simulink model "test_emplanner_cs"  (R2021a)
settings: Solver=ode5  StartTime=0.0  StopTime=120  FixedStep=1/1000  RelTol=1e-3
PreLoadFcn:
  | mbxruntime.callbacks.PreLoadFcn(bdroot);
PostLoadFcn:
  | mbxruntime.callbacks.PostLoadFcn(bdroot);
InitFcn:
  | mbxruntime.callbacks.InitFcn(bdroot);
StartFcn:
  | mbxruntime.callbacks.StartFcn(bdroot);
StopFcn:
  | mbxruntime.callbacks.StopFcn(bdroot);
model workspace (MAT data in the model file):
  mbox_table : object (value not decoded)
  model_closed = 0
  sim_status = 0
values from neighbouring files (symbols this model uses):
  c_factor = 43.75    [emplanner_init.m]
  cf = -175016    [emplanner_init.m]
  cr = -130634    [emplanner_init.m]
  global_path_x = [-2.7494 -1.75001774493 -0.751894634419 0.244952249347 1.24051712279 2.23479835808 3.22779585569 4.21951007764 5.20994169183 6.19909144113 7.18696009523 8.17354843293 ... (3001 elements, 3001x1)]    [global_path.mat]
  global_path_y = [18.2589 18.2589 18.2589 18.2589 18.2589 18.2589 18.2589 18.2589 18.2589 18.2589 18.2589 18.2589 ... (3001 elements, 3001x1)]    [global_path.mat]
  KD_PID_distance = 0.0    (= 0)    [emplanner_init.m]
  KD_PID_speed = 0    [emplanner_init.m]
  KI_PID_distance = 0.0    (= 0)    [emplanner_init.m]
  KI_PID_speed = 0    [emplanner_init.m]
  KP_PID_distance = 0.5    [emplanner_init.m]
  KP_PID_speed = 1.8    [emplanner_init.m]
  la = 1.265    [emplanner_init.m]
  lb = 2.947-1.265    (= 1.682)    [emplanner_init.m]
  LQR_K1 = k(:,1)'    [emplanner_init.m]
  LQR_K2 = k(:,2)'    [emplanner_init.m]
  LQR_K3 = k(:,3)'    [emplanner_init.m]
  LQR_K4 = k(:,4)'    [emplanner_init.m]
  m = 2020    [emplanner_init.m]
  rack_displacement = [-39.14 , -37.2 , -35.29 , -33.43 , -31.6 , -29.81 , -28.06 , -26.34 , -24.66 ,      -23.01 , -21.38 , -19.79 , -18.23 , -16.69 , -15.18 , -13.7 , -12.23 , -10.8 , -9.38 , -7.98 ,     -6.61 , -5.25 , -3.91 , -2.59 , -1.29 , 0 , 1.27 , 2.54 , 3.78 , 5.02 , 6.24 , 7.46 , 8.66 ,      9.86 , 11.05 , 12.24 , 13.41 , 14.59 , 15.76 , 16.92 , 18.09 , 19.25 , 20.42 , 21.59 , 22.76 ,      23.93 , 25.11 , 26 ...(+26 chars)    [emplanner_init.m]
  right_wheel_ground = [-70 ,-67.2 , -64.4 , -61.6 , -58.8 , -56 , -53.2 , -50.4 , -47.6 , -44.8 , -42 ,      -39.2 , -36.4 , -33.6 , -30.8 , -28 , -25.2 , -22.4 , -19.6 , -16.8 , -14 , -11.2 , -8.4 , -5.6 ,      -2.8 , 0 , 2.8 , 5.6 , 8.4 , 11.2 , 14 , 16.8 , 19.6 , 22.4 , 25.2 , 28 , 30.8 , 33.6 , 36.4 ,      39.2 , 42 , 44.8 , 47.6 , 50.4 , 53.2 , 56 , 58.8 , 61.6 , 64.4 , 67.2 , 70 ]    [emplanner_init.m]
  vx_break_point = zeros(1,5000)    [emplanner_init.m]
undefined symbols (not defined in the file or in its folder): aubr, DiscIntNeverNeededParam, tablebr, vubr, warningInitialVelocity, x0
libraries: PreScanSimulinkLibrary x27, simulink x19, simulink_extras x6, Solver_SF x1
(part 10 of 11)

== matlab function test_emplanner_cs/Audi_A8_Sedan_1/decision&planning module/EM Planner/obs/cartesian2frenet1/MATLAB Function1 ==
  data: x_set input; s_set output; y_set input; frenet_path_x input; frenet_path_y input; proj_x_set input; proj_y_set input; proj_heading_set input; proj_match_point_index_set input; index2s input; l_set output
function [s_set,l_set] = fcn(x_set,y_set,frenet_path_x,frenet_path_y,...
    proj_x_set,proj_y_set,proj_heading_set,proj_match_point_index_set,index2s)
%该函数计算世界坐标系下的x_set,y_set的点转换到frenet_path下的坐标s l
%输入： x_set,y_set待坐标转换的点
    %  frenet_path_x,frenet_path_y  frenet坐标轴
    %  proj_x,y,heading,kappa,index 待坐标转换点的投影点的信息
    %  inde2s  frenet_path的index与s的转换表
    n=128;
    s_set=ones(n,1)*nan;
    l_set=ones(n,1)*nan;
    for i=1:length(x_set)
        if isnan(x_set(i))
            break;
        end
        s_set(i)=CalSFormIndex2S(index2s,frenet_path_x,frenet_path_y,...
            proj_x_set(i),proj_y_set(i),proj_match_point_index_set(i));
        n_r=[-sin(proj_heading_set(i));cos(proj_heading_set(i))];
        r_h=[x_set(i);y_set(i)];
        r_r=[proj_x_set(i);proj_y_set(i)];
        l_set(i)=(r_h-r_r)'*n_r;
    end
end

function s=CalSFormIndex2S(index2s,path_x,path_y,proj_x,proj_y,proj_match_point_index)
    %该函数将计算给定index2s的映射关系后，计算点（proj_x,proj_y）所对应的弧长
    %投影点与匹配点的误差向量
    vector_1=[proj_x;proj_y]-[path_x(proj_match_point_index);path_y(proj_match_point_index)];
    if proj_match_point_index<length(path_x)
        %匹配点切线处的方向向量
        vector_2=[path_x(proj_match_point_index+1);path_y(proj_match_point_index+1)]-...
            [path_x(proj_match_point_index);path_y(proj_match_point_index)];
    else
         vector_2=[path_x(proj_match_point_index);path_y(proj_match_point_index)]-...
            [path_x(proj_match_point_index-1);path_y(proj_match_point_index-1)];
    end
    if vector_1'*vector_2>0
        %投影点在匹配点前面
        s=index2s(proj_match_point_index)+sqrt(vector_1'*vector_1);
    else
        %投影点在匹配点后面
        s=index2s(proj_match_point_index)-sqrt(vector_1'*vector_1);
    end
end

== matlab function test_emplanner_cs/Audi_A8_Sedan_1/decision&planning module/EM Planner/qp ==
  data: qp_path_s output; l_min input; qp_path_l output; l_max input; w_cost_l input; w_cost_dl input; w_cost_ddl input; w_cost_dddl input; w_cost_centre input; w_cost_end_l input; w_cost_end_dl input; w_cost_end_ddl input; host_d1 input; host_d2 input; host_w input; plan_start_s input; plan_start_l input; plan_start_dl input; plan_start_ddl input; qp_path_dl output; qp_path_ddl output; delta_dl_max input; delta_ddl_max input
function [qp_path_s,qp_path_l,qp_path_dl,qp_path_ddl] = ...
    fcn(l_min,l_max,w_cost_l,w_cost_dl,w_cost_ddl,w_cost_dddl,w_cost_centre,w_cost_end_l,w_cost_end_dl,w_cost_end_ddl,...
    host_d1,host_d2,host_w,...
    plan_start_s,plan_start_l,plan_start_dl,plan_start_ddl,...
    delta_dl_max,delta_ddl_max)
%路径二次规划
%输入:l_min,l_max点的凸空间
%   参考线代价：w_cost_l
%   光滑性代价：w_cost_dl,ddl,dddl
%   凸空间中央代价：w_cost_centre
%   w_cost_end_l,dl,ddl终点的状态代价（希望path的终点状态为（0，0，0））
%   host_d1,d2 代表质心到车头尾的距离
%   host_w 为host的宽度
%   plan_start_l,dl,ddl 规划起点状态
%输出：qp_path_l,dl,ddl 二次规划的曲线
coder.extrinsic("quadprog");
n=20;
%输出初始化
qp_path_s=zeros(n,1);
qp_path_l=zeros(n,1);
qp_path_dl=zeros(n,1);
qp_path_ddl=zeros(n,1);
H_L=zeros(3*n,3*n);
H_DL=zeros(3*n,3*n);
H_DDL=zeros(3*n,3*n);
H_DDDL=zeros(n-1,3*n);
H_L_END=zeros(3*n,3*n);
H_DL_END=zeros(3*n,3*n);
H_DDL_END=zeros(3*n,3*n);
Aeq=zeros(2*n-2,3*n);
beq=zeros(2*n-2,1);
A=zeros(8*n,3*n);
b=zeros(8*n,1);
%更新加入dl(i+1)-dl(i)ddl(i+1)-ddl(i)的约束
A_dl_minus=zeros(n-1,3*n);
b_dl_minus=zeros(n-1,1);
A_ddl_minus=zeros(n-1,3*n);
b_ddl_minus=zeros(n-1,1);
for i=1:n-1
    row=i;
    col=3*i-2;
    A_dl_minus(row,col:col+5)=[0 -1 0 0 1 0];
    b_dl_minus(row)=delta_dl_max;
    A_ddl_minus(row,col:col+5)=[0 0 -1 0 0 1];
    b_ddl_minus(row)=delta_ddl_max;
end
A_minus=[A_dl_minus;
         -A_dl_minus;
         A_ddl_minus;
         -A_ddl_minus;];
b_minus=[b_dl_minus;
         b_dl_minus;
         b_ddl_minus;
         b_ddl_minus;];
%期望终点状态
end_l_desire=0;
end_dl_desire=0;
end_ddl_desire=0;
%Aeq_sub
ds=3;%纵向间隔
for i=1:n
    qp_path_s(i)=plan_start_s+(i-1)*ds;
end
Aeq_sub=[1 ds ds^2/3 -1 0 ds^2/6;
        0 1 ds/2 0 -1 ds/2];
%A_sub
d1=host_d1;
d2=host_d2;
w=host_w;
A_sub=[1 d1 0;
       1 d1 0;
       1 -d2 0;
       1 -d2 0;
       -1 -d1 0;
       -1 -d1 0;
       -1 d2 0;
       -1 d2 0];
%生成Aeq
for i=1:n-1
    %计算分块矩阵左上角的行和列
    row=2*i-1;
    col=3*i-2;
    Aeq(row:row+1,col:col+5)=Aeq_sub;
end
%生成A
for i=2:n
    row=8*i-7;
    col=3*i-2;
    A(row:row+7,col:col+2)=A_sub;
end
%生成b
%找到四个角点所对应的l_min,l_max即可
front_index=ceil(d1/ds);
back_index=ceil(d2/ds);
for i=2:n
    %左前 右前的index=min(i+front_index,60)
    %左后 右后的index=max(i-back_index,1)
    index1=min(3*i-2+front_index,n);
    index2=max(3*i-2-back_index,1);
    b(8*i-7:8*i,1)=[l_max(index1)-w/2;
                    l_max(index1)+w/2;
                    l_max(index2)-w/2;
                    l_max(index2)+w/2;
                    -l_min(index1)+w/2;
                    -l_min(index1)-w/2;
                    -l_min(index2)+w/2;
                    -l_min(index2)-w/2;];
end
%生成lb ub 主要是对规划起点进行约束
lb=ones(3*n,1)*-inf;
ub=ones(3*n,1)*inf;
lb(1)=plan_start_l;
lb(2)=plan_start_dl;
lb(3)=plan_start_ddl;
ub(1)=lb(1);
ub(2)=lb(2);
ub(3)=lb(3);
for i=2:n
    lb(3*i-1)=-2;%约束l'
    ub(3*i-1)=2;
    lb(3*i)=-0.1;%约束l''
    ub(3*i)=0.1;
end
%生成H_L,H_DL,H_DDL,H_CENTRE
for i=1:n
    H_L(3*i-2,3*i-2)=1;
    H_DL(3*i-1,3*i-1)=1;
    H_DDL(3*i,3*i)=1;
end
H_CENTRE=H_L;
%生成H_DDDL
H_dddl_sub=[0 0 1 0 0 -1];
for i=1:n-1
    row=i;
    col=3*i-2;
    H_DDDL(row,col:col+5)=H_dddl_sub;
end
%生成H_L_END,H_DL_END,H_DDL_END
H_L_END(3*n-2,3*n-2)=1;
H_DL_END(3*n-1,3*n-1)=1;
H_DDL_END(3*n,3*n)=1;
%生成二次规划的H
H=w_cost_l*(H_L'*H_L)+w_cost_dl*(H_DL'*H_DL)+w_cost_ddl*(H_DDL'*H_DDL)+...
    w_cost_dddl*(H_DDDL'*H_DDDL)/ds+w_cost_centre*(H_CENTRE'*H_CENTRE)+w_cost_end_l*(H_L_END'*H_L_END)+...
    w_cost_end_dl*(H_DL_END'*H_DL_END)+w_cost_end_ddl*(H_DDL_END'*H_DDL_END);
H=2*H;
%生成f
f=zeros(3*n,1);
centre_line=0.5*(l_min+l_max);%此时centre line还是60个点
% centre_line=dp_path_l_final;
%尽可能靠近centre_line
for i=1:n
    f(3*i-2)=-2*centre_line(3*i-2);
end
%避免centreline权重过大影响轨迹平顺性
for i=1:n
    if abs(f(i))>0.3
        f(i)=w_cost_centre*f(i);
    end
end
%终点要接近end_l dl ddl desire
f(3*n-2)=f(3*n-2)-2*end_l_desire*w_cost_end_l;
f(3*n-1)=f(3*n-1)-2*end_dl_desire*w_cost_end_dl;
f(3*n)=f(3*n)-2*end_ddl_desire*w_cost_end_ddl;

X=quadprog(H,f,A,b,Aeq,beq,lb,ub);
%这里没有对曲率做约束
for i=1:n
    qp_path_l(i)=X(3*i-2);
    qp_path_dl(i)=X(3*i-1);
    qp_path_ddl(i)=X(3*i);
end
end

== matlab function test_emplanner_cs/Audi_A8_Sedan_1/decision&planning module/EM Planner/plot ==
  data: dp_s input; dp_l input; qp_s input; qp_l input; l_min input; l_max input; obs_s_set input; obs_l_set input; start_s input; start_l input; start_dl input
function  fcn(dp_s,dp_l,qp_s,qp_l,l_min,l_max,obs_s_set,obs_l_set,start_s,start_l,start_dl)
coder.extrinsic("plot","axis","figure","drawnow","cla","fill");

obs_length = 5;
obs_width = 2;
host_l = 6;
host_w = 1.63;
cla;
host_p1_l = start_l + sin(atan(start_dl)) * host_l /2 + host_w/2 * cos(atan(start_dl));
host_p1_s = start_s + cos(atan(start_dl)) * host_l /2 - host_w/2 * sin(atan(start_dl));
host_p2_l = start_l + sin(atan(start_dl)) * host_l /2 - host_w/2 * cos(atan(start_dl));
host_p2_s = start_s + cos(atan(start_dl)) * host_l /2 + host_w/2 * sin(atan(start_dl));
host_p3_l = start_l - sin(atan(start_dl)) * host_l /2 + host_w/2 * cos(atan(start_dl));
host_p3_s = start_s - cos(atan(start_dl)) * host_l /2 - host_w/2 * sin(atan(start_dl));
host_p4_l = start_l - sin(atan(start_dl)) * host_l /2 - host_w/2 * cos(atan(start_dl));
host_p4_s = start_s - cos(atan(start_dl)) * host_l /2 + host_w/2 * sin(atan(start_dl));
host_area_x = [host_p1_s;host_p2_s;host_p4_s;host_p3_s];
host_area_y = [host_p1_l;host_p2_l;host_p4_l;host_p3_l];
fill(host_area_x,host_area_y,[0 1 1]);
hold on
plot(dp_s,dp_l,'r');

plot(qp_s,qp_l,'b');
plot(dp_s,l_min,dp_s,l_max);
axis([-8 70 -10 10]);

for i = 1:length(obs_s_set)
    if isnan(obs_s_set(i))
        break;
    end
    obs_p1_s = obs_s_set(i) + obs_length/2;
    obs_p1_l = obs_l_set(i) + obs_width/2;
    obs_p2_s = obs_s_set(i) + obs_length/2;
    obs_p2_l = obs_l_set(i) - obs_width/2;
    obs_p3_s = obs_s_set(i) - obs_length/2;
    obs_p3_l = obs_l_set(i) + obs_width/2;
    obs_p4_s = obs_s_set(i) - obs_length/2;
    obs_p4_l = obs_l_set(i) - obs_width/2;
    obs_area_s = [obs_p1_s;obs_p2_s;obs_p4_s;obs_p3_s];
    obs_area_l = [obs_p1_l;obs_p2_l;obs_p4_l;obs_p3_l];
    fill(obs_area_s,obs_area_l,[0 0 0]);
end

== matlab function test_emplanner_cs/Audi_A8_Sedan_1/decision&planning module/EM Planner/MATLAB Function2 ==
  data: trajectory_heading_final input; y output
function y = fcn(trajectory_heading_final)
y = zeros(421,1);
y(1) = trajectory_heading_final(1);
for i = 2:421
    y(i) = y(i-1) + sin(trajectory_heading_final(i) - trajectory_heading_final(i-1));
end

== matlab function test_emplanner_cs/Audi_A8_Sedan_1/decision&planning module/EM Planner/obs/cartesian2frenet1/MATLAB Function2 ==
  data: ax_set input; s_dot2_set output; ay_set input; proj_heading_set input; proj_kappa_set input; l_set input; s_dot_set input; dl_set input; l_dot2_set output; ddl_set output
function [s_dot2_set,l_dot2_set,ddl_set] = fcn(ax_set,ay_set,proj_heading_set,proj_kappa_set,l_set,s_dot_set,dl_set)
n=128;
s_dot2_set=ones(n,1)*nan;
l_dot2_set=ones(n,1)*nan;
ddl_set=ones(n,1)*nan;
for i=1:length(l_set)
    if isnan(l_set(i))
        break;
    end
    a_h=[ax_set(i);ay_set(i)];
    n_r=[-sin(proj_heading_set(i));cos(proj_heading_set(i))];
    t_r=[cos(proj_heading_set(i));sin(proj_heading_set(i))];
    %近似认为dkr/ds为0，简化计算
    s_dot2_set(i)=(a_h'*t_r)/(1-proj_kappa_set(i)*l_set(i))+(proj_kappa_set(i)*(s_dot_set(i)^2)*dl_set)/(1-proj_kappa_set(i)*l_set(i))+...
        (s_dot_set(i)^2)*(proj_kappa_set(i)*dl_set(i))/(1-proj_kappa_set(i)*l_set(i));
    l_dot2_set(i)=a_h'*n_r-proj_kappa_set(i)*(1-proj_kappa_set(i)*l_set(i))*(s_dot_set(i)^2);
    %考虑加速度为0的情况
    if s_dot_set(i)<1e-6
        ddl_set(i)=0;
    else
        ddl_set(i)=(l_dot2_set(i)-dl_set(i)*s_dot2_set(i))/(s_dot_set(i)^2);
    end
end

== matlab function test_emplanner_cs/Audi_A8_Sedan_1/decision&planning module/EM Planner/obs/MATLAB Function ==
  data: obs_x_set_gcs input; static_obs_x_set output; obs_y_set_gcs input; obs_heading_set_gcs input; obs_velocity_set_gcs input; static_obs_y_set output; dynamic_obs_x_set output; dynamic_obs_y_set output; dynamic_obs_vx_set output; dynamic_obs_vy_set output
function [static_obs_x_set,static_obs_y_set,dynamic_obs_x_set,dynamic_obs_y_set,dynamic_obs_vx_set,dynamic_obs_vy_set] ...
    = fcn(obs_x_set_gcs,obs_y_set_gcs,obs_heading_set_gcs,obs_velocity_set_gcs)
    %该函数分类静态障碍物和动态障碍物
n=32;
static_obs_x_set=ones(n,1)*nan;
static_obs_y_set=ones(n,1)*nan;
dynamic_obs_x_set=ones(n,1)*nan;
dynamic_obs_y_set=ones(n,1)*nan;
dynamic_obs_vx_set=ones(n,1)*nan;
dynamic_obs_vy_set=ones(n,1)*nan;
count_static=1;
count_dynamic=1;
for i=1:length(obs_x_set_gcs)
    if isnan(obs_x_set_gcs(i))
        break;
    end
    if abs(obs_velocity_set_gcs(i))<0.1
        static_obs_x_set(count_static)=obs_x_set_gcs(i);
        static_obs_y_set(count_static)=obs_y_set_gcs(i);
        count_static=count_static+1;
    else
        dynamic_obs_x_set(count_dynamic)=obs_x_set_gcs(i);
        dynamic_obs_y_set(count_dynamic)=obs_y_set_gcs(i);
        dynamic_obs_vx_set(count_dynamic) = obs_velocity_set_gcs(i)*cos(obs_heading_set_gcs(i));
        dynamic_obs_vy_set(count_dynamic) = obs_velocity_set_gcs(i)*sin(obs_heading_set_gcs(i));
        count_dynamic=count_dynamic+1;
    end
end

== matlab function test_emplanner_cs/Audi_A8_Sedan_1/decision&planning module/EM Planner/path desion with dynamic planning(dp) ==
  data: obs_s_set input; dp_path_s output; obs_l_set input; plan_start_s input; plan_start_l input; plan_start_dl input; plan_start_dll input; w_cost_collision input; w_cost_smooth_dl input; w_cost_smooth_ddl input; w_cost_smooth_dddl input; w_cost_ref input; row input; col input; sample_s input; sample_l input; dp_path_l output
function [dp_path_s,dp_path_l] = fcn(obs_s_set,obs_l_set,plan_start_s,plan_start_l,plan_start_dl,plan_start_dll,...
    w_cost_collision,w_cost_smooth_dl,w_cost_smooth_ddl,w_cost_smooth_dddl,w_cost_ref,row,col,sample_s,sample_l)
%路径动态规划主函数
%输入： obs s l set 筛选后障碍物的sl信息
%       plan_start s l dl ddl 规划起点信息
%       w_cost...动态规划代价权重
%       sample_s,sample_l 采样的s l长度
%输出： dp_path_l,dp_path_s 动态规划的路径s l,此路径不包含规划起点
%声明二维矩阵变量node_cost(i,j),node_cost(i,j)表示从起点出发，到行i列j节点的最小代价
node_cost=ones(row,col)*inf;%初始化为无穷大
%声明二维矩阵变量pre_node_index
%pre_node_index(i,j)表示从起点到i行j列的最优路径前一节点的行号，因为如果第n个节点前一个列号为n-1已知
pre_node_index=zeros(row,col);%初始化，默认所有节点的最优节点行号都是0，即为起点
%计算从起点到第一列的cost
for i=1:row
    node_cost(i,1)=CalcStartCost(plan_start_s,plan_start_l,plan_start_dl,plan_start_dll,i,sample_s,sample_l,...
    w_cost_collision,w_cost_smooth_dl,w_cost_smooth_ddl,w_cost_smooth_dddl,w_cost_ref,obs_s_set,obs_l_set,row);
end
%动态规划主函数，从第二列开始
for j=2:col
    for i=1:row
        %计算当前node(i,j)的s,l
        cur_node_s=plan_start_s+(j)*sample_s;
        cur_node_l=((row+1)/2-i)*sample_l;
        %遍历前一列的节点
        for k=1:row
            %计算前一列节点的s,l
            pre_node_s=plan_start_s+(j-1)*sample_s;
            pre_node_l=((row+1)/2-k)*sample_l;
            cost_neighbour=CalaNeigbourCost(pre_node_s,pre_node_l,cur_node_s,cur_node_l,...
            w_cost_collision,w_cost_smooth_dl,w_cost_smooth_ddl,w_cost_smooth_dddl,w_cost_ref,obs_s_set,obs_l_set);
            %起点到上一个节点的最小代价为node_cost(k,j-1)
            pre_min_cost=node_cost(k,j-1);
            %起点到node_cost(i,j)的最小代价为node_cost(k,j-1)加上node(k,j-1)到node(i,j)的代价（k=1,2...row）中最小的
            cost_temp=pre_min_cost+cost_neighbour;
            if cost_temp<node_cost(i,j)
                node_cost(i,j)=cost_temp;
                %把最优路径上一列节点的行号记录下来
                pre_node_index(i,j)=k;
            end
        end
    end
end
%找到node_cost最后一列中，cost最小的，记代价最小的行号为index
index=0;
min_cost=inf;
for i=1:row
    if node_cost(i,end)<min_cost
        min_cost=node_cost(i,end)
        index=i;
    end
end
%动态规划最优路径初始化
dp_node_list_row=zeros(col,1);
%从后往前递推
cur_index=index;
for i=1:col
    pre_index=pre_node_index(cur_index,end-i+1);
    dp_node_list_row(col-i+1)=cur_index;
    cur_index=pre_index;
end
%输出初始化
dp_path_s=ones(15,1)*-1;
dp_path_l=ones(15,1)*-1;
for i=1:col
    dp_path_s(i)=plan_start_s+i*sample_s;
    dp_path_l(i)=((row+1)/2-dp_node_list_row(i))*sample_l;
end

end

function cost=CalaNeigbourCost(pre_node_s,pre_node_l,cur_node_s,cur_node_l,...
            w_cost_collision,w_cost_smooth_dl,w_cost_smooth_ddl,w_cost_smooth_dddl,w_cost_ref,obs_s_set,obs_l_set)
        %该函数将计算相邻两个节点的cost
    start_l=pre_node_l;
    start_dl=0;
    start_ddl=0;
    end_l=cur_node_l;
    end_dl=0;
    end_ddl=0;
    start_s=pre_node_s;
    end_s=cur_node_s;
    coeff=CalQuinticCoeffient(start_l,start_dl,start_ddl,end_l,end_dl,end_ddl,start_s,end_s);
    a0=coeff(1);
    a1=coeff(2);
    a2=coeff(3);
    a3=coeff(4);
    a4=coeff(5);
    a5=coeff(6);
    %取10个点计算cost
    ds=zeros(10,1);
    l=zeros(10,1);
    dl=zeros(10,1);
    ddl=zeros(10,1);
    dddl=zeros(10,1);
    for j=1:10
        ds(j)=start_s+(j-1)*(end_s-start_s)/10; 
    end
    l=a0*ones(10,1)+a1*ds+a2*ds.^2+a3*ds.^3+a4*ds.^4+a5*ds.^5;
    dl=a1*ones(10,1)+2*a2*ds+3*a3*ds.^2+4*a4*ds.^3+5*a5*ds.^4;
    ddl=2*a2*ones(10,1)+6*a3*ds+12*a4*ds.^2+20*a5*ds.^3;
    dddl=6*a3*ones(10,1)+24*a4*ds+60*a5*ds.^2;
    cost_smooth=w_cost_smooth_dl*(dl'*dl)+w_cost_smooth_ddl*(ddl'*ddl)+w_cost_smooth_dddl*(dddl'*dddl);
    cost_ref=w_cost_ref*(l'*l);
    cost_collision=0;
    for i=1:length(obs_s_set)
        if isnan(obs_s_set(i))
            break;
        end
        dlon=ones(10,1)*obs_s_set(i)-ds;
        dlat=ones(10,1)*obs_l_set(i)-l;
        %这里做了简化模型，认为障碍物为一个点
        square_d=dlon.^2+dlat.^2;
        cost_collision_once=CalcObsCost(w_cost_collision,square_d);
        cost_collision=cost_collision+cost_collision_once;
    end
    cost=cost_collision+cost_smooth+cost_ref; 
end

function cost=CalcStartCost(begin_s,begin_l,begin_dl,begin_ddl,cur_node_row,sample_s,sample_l,...
    w_cost_collision,w_cost_smooth_dl,w_cost_smooth_ddl,w_cost_smooth_dddl,w_cost_ref,obs_s_set,obs_l_set,row)
%该函数计算起点到第一层的cost
    start_l=begin_l;
    start_dl=begin_dl;
    start_ddl=begin_ddl;
    end_l=((row+1)/2-cur_node_row)*sample_l;
    end_dl=0;
    end_ddl=0;
    start_s=begin_s;
    end_s=begin_s+sample_s;
    coeff=CalQuinticCoeffient(start_l,start_dl,start_ddl,end_l,end_dl,end_ddl,start_s,end_s);
    a0=coeff(1);
    a1=coeff(2);
    a2=coeff(3);
    a3=coeff(4);
    a4=coeff(5);
    a5=coeff(6);
    %取10个点计算cost
    ds=zeros(10,1);
    l=zeros(10,1);
    dl=zeros(10,1);
    ddl=zeros(10,1);
    dddl=zeros(10,1);
    for j=1:10
        ds(j)=start_s+(j-1)*sample_s/10; 
    end
    l=a0*ones(10,1)+a1*ds+a2*ds.^2+a3*ds.^3+a4*ds.^4+a5*ds.^5;
    dl=a1*ones(10,1)+2*a2*ds+3*a3*ds.^2+4*a4*ds.^3+5*a5*ds.^4;
    ddl=2*a2*ones(10,1)+6*a3*ds+12*a4*ds.^2+20*a5*ds.^3;
    dddl=6*a3*ones(10,1)+24*a4*ds+60*a5*ds.^2;
    cost_smooth=w_cost_smooth_dl*(dl'*dl)+w_cost_smooth_ddl*(ddl'*ddl)+w_cost_smooth_dddl*(dddl'*dddl);
    cost_ref=w_cost_ref*(l'*l);
    cost_collision=0;
    for i=1:length(obs_s_set)
        if isnan(obs_s_set(i))
            break;
        end
        dlon=ones(10,1)*obs_s_set(i)-ds;
        dlat=ones(10,1)*obs_l_set(i)-l;
        %这里做了简化模型，认为障碍物为一个点
        square_d=dlon.^2+dlat.^2;
        cost_collision_once=CalcObsCost(w_cost_collision,square_d);
        cost_collision=cost_collision+cost_collision_once;
    end
    cost=cost_collision+cost_smooth+cost_ref;
end

function obs_cost=CalcObsCost(w_cost_collision,square_d)
%该函数计算障碍物的距离代价
%超过4米的cost为0 在4到3米的cost为1000/squard_d,在小于3米cost为w_cost_collision
    cost=0;
    for i=1:length(square_d)
        if(square_d(i)<16&&square_d(i)>9)
            cost=cost+1000/square_d(i);
        elseif (square_d(i)<9)
            cost=cost+w_cost_collision;
        end
    end
    obs_cost=cost;
end
function coeff=CalQuinticCoeffient(start_l,start_dl,start_ddl,end_l,end_dl,end_ddl,start_s,end_s)
    start_s2=start_s*start_s;
    start_s3=start_s2*start_s;
    start_s4=start_s3*start_s;
    start_s5=start_s4*start_s;
    end_s2=end_s*end_s;
    end_s3=end_s2*end_s;
    end_s4=end_s3*end_s;
    end_s5=end_s4*end_s;
    A=[1,start_s,start_s2, start_s3,  start_s4,   start_s5;
       0 1,      2*start_s,3*start_s2,4*start_s3, 5*start_s4;
       0 0,      2,        6*start_s, 12*start_s2,20*start_s3;
       1,end_s,  end_s2,   end_s3,    end_s4,     end_s5;
       0 1,      2*end_s,  3*end_s2,  4*end_s3,   5*end_s4;
       0 0,      2,        6*end_s,   12*end_s2,  20*end_s3;];
   B=[start_l;
       start_dl;
       start_ddl;
       end_l;
       end_dl;
       end_ddl;];
   coeff=A\B;
end

== matlab function test_emplanner_cs/Audi_A8_Sedan_1/decision&planning module/EM Planner/increase DP path nodes ==
  data: dp_path_s_init input; dp_path_s_final output; dp_path_l_init input; plan_start_s input; plan_start_l input; plan_start_dl input; plan_start_ddl input; dp_path_l_final output; dp_path_dl_final output; dp_path_ddl_final output
function [dp_path_s_final,dp_path_l_final,dp_path_dl_final,dp_path_ddl_final] = ...
    fcn(dp_path_s_init,dp_path_l_init,plan_start_s,plan_start_l,plan_start_dl,plan_start_ddl)
%该函数增密dp_path_s,dp_path_l
%动态规划的行和列未知
%每1“米”采样一个，一共60个
ds=1;
dp_path_s_final=ones(60,1)*nan;
dp_path_l_final=ones(60,1)*nan;
dp_path_dl_final=ones(60,1)*nan;
dp_path_ddl_final=ones(60,1)*nan;

%设置五次多项式的起点
start_s=plan_start_s;
start_l=plan_start_l;
start_dl=plan_start_dl;
start_ddl=plan_start_ddl;

s_cur=[];
l_temp=[];
dl_temp=[];
ddl_temp=[];
for i=1:length(dp_path_s_init)
    if dp_path_s_init(i)==-1
        break;
    end
    for j=1:10000
        s_node=start_s+ds*(j-1);
        if s_node<dp_path_s_init(i)
            s_cur=[s_cur,s_node];
        else
            break;
        end
    end
    end_s=dp_path_s_init(i);
    end_l=dp_path_l_init(i);
    end_dl=0;
    end_ddl=0;
    coeff=CalQuinticCoeffient(start_l,start_dl,start_ddl,end_l,end_dl,end_ddl,start_s,end_s);
    a0=coeff(1);
    a1=coeff(2);
    a2=coeff(3);
    a3=coeff(4);
    a4=coeff(5);
    a5=coeff(6);
    l=a0*ones(1,length(s_cur))+a1*s_cur+a2*s_cur.^2+a3*s_cur.^3+...
        a4*s_cur.^4+a5*s_cur.^5;
    dl=a1*ones(1,length(s_cur))+2*a2*s_cur+3*a3*s_cur.^2+...
        4*a4*s_cur.^3+5*a5*s_cur.^4;
    ddl=2*a2*ones(1,length(s_cur))+6*a3*s_cur+12*a4*s_cur.^2+...
        20*a5*s_cur.^3;
    l_temp=[l_temp,l];
    dl_temp=[dl_temp,dl];
    ddl_temp=[ddl_temp,ddl];
    start_s=end_s;
    start_l=end_l;
    start_dl=end_dl;
    start_ddl=end_ddl;
    s_cur=[];
end
    for k=1:length(l_temp)
        if k==61
            break;
        end
        dp_path_s_final(k)=plan_start_s+ds*(k-1);
        dp_path_l_final(k)=l_temp(k);
        dp_path_dl_final(k)=dl_temp(k);
        dp_path_ddl_final(k)=ddl_temp(k);
    end
end

function coeff=CalQuinticCoeffient(start_l,start_dl,start_ddl,end_l,end_dl,end_ddl,start_s,end_s)
    start_s2=start_s*start_s;
    start_s3=start_s2*start_s;
    start_s4=start_s3*start_s;
    start_s5=start_s4*start_s;
    end_s2=end_s*end_s;
    end_s3=end_s2*end_s;
    end_s4=end_s3*end_s;
    end_s5=end_s4*end_s;
    A=[1,start_s,start_s2, start_s3,  start_s4,   start_s5;
       0,1,      2*start_s,3*start_s2,4*start_s3, 5*start_s4;
       0,0,      2,        6*start_s, 12*start_s2,20*start_s3;
       1,end_s,end_s2, end_s3,  end_s4,   end_s5;
       0,1,    2*end_s,3*end_s2,4*end_s3, 5*end_s4;
       0,0,    2,      6*end_s, 12*end_s2,20*end_s3;];
   B=[start_l;
       start_dl;
       start_ddl;
       end_l;
       end_dl;
       end_ddl;];
   coeff=A\B;
end

== matlab function test_emplanner_cs/Audi_A8_Sedan_1/decision&planning module/EM Planner/ frenet2cartesian ==
  data: s_set input; x_set output; l_set input; dl_set input; ddl_set input; frenet_path_x input; frenet_path_y input; frenet_path_heading input; frenet_path_kappa input; index2s input; y_set output; heading_set output; kappa_set output
function [x_set,y_set,heading_set,kappa_set] = ...
    fcn(s_set,l_set,dl_set,ddl_set,frenet_path_x,frenet_path_y,frenet_path_heading,frenet_path_kappa,index2s)
    %通用算法 frenet转frenet
    x_set=ones(600,1)*nan;
    y_set=ones(600,1)*nan;
    heading_set=ones(600,1)*nan;
    kappa_set=ones(600,1)*nan;
    for i=1:length(s_set)
        if isnan(s_set(i))
            break;
        end
        [proj_x,proj_y,proj_heading,proj_kappa]=CalProjPoint(s_set(i),frenet_path_x,frenet_path_y,frenet_path_heading...
    ,frenet_path_kappa,index2s)
        nor=[-sin(proj_heading);cos(proj_heading)];
        tor=[cos(proj_heading);sin(proj_heading)];
        point=[proj_x;proj_y]+l_set(i)*nor;
        x_set(i)=point(1);
        y_set(i)=point(2);
        heading_set(i)=proj_heading+atan(dl_set(i)/(1-proj_kappa*l_set(i)));
        %近似认为kappa'=0
        kappa_set(i)=((ddl_set(i)+proj_kappa*dl_set(i)*tan(heading_set(i)-proj_heading))*...
            (cos(heading_set(i)-proj_heading)^2 )/(1-proj_kappa*l_set(i))+proj_kappa)*...
            cos(heading_set(i)-proj_heading)/(1-proj_kappa*l_set(i));
    end
end


function [proj_x,proj_y,proj_heading,proj_kappa]=CalProjPoint(s,frenet_path_x,frenet_path_y,frenet_path_heading...
    ,frenet_path_kappa,index2s)
%该函数计算在frenet坐标系，点（s,l）在frenet坐标轴的投影的直角坐标
    match_index=1;
    while index2s(match_index)<s
        match_index=match_index+1;
    end
    match_point=[frenet_path_x(match_index);frenet_path_y(match_index)];
    match_point_heading=frenet_path_heading(match_index);
    match_point_kappa=frenet_path_kappa(match_index);
    ds=s-index2s(match_index);
    match_tor=[cos(match_point_heading);sin(match_point_heading)];
    proj_point=match_point+ds*match_tor;
    proj_heading=match_point_heading+ds*match_point_kappa;
    proj_kappa=match_point_kappa;
    proj_x=proj_point(1);
    proj_y=proj_point(2);
end

== matlab function test_emplanner_cs/Audi_A8_Sedan_2/PathFollower_Preview_1/LateralController/CTRL REFERENCES/Calculate Lateral Error/eml_find_10k_lateral_error_points ==
  data: pvp input size=2; dist_psvehicle output size=10; TrajOffset_x_y_Y input size=3; ActorOffset_Left_Right input; p0 input size=2; PreviewDistance input size=10; Traj_x parameter; Traj_y parameter; Traj_t parameter; Traj_v parameter; RefreshCounter parameter
function dist_psvehicle  = eml_find_10k_lateral_error_points(pvp,TrajOffset_x_y_Y,ActorOffset_Left_Right,p0,PreviewDistance,Traj_x,Traj_y,Traj_t,Traj_v,RefreshCounter)

dist_psvehicle = emlfcn_find_10k_lateral_error_points(pvp,TrajOffset_x_y_Y,ActorOffset_Left_Right,p0,PreviewDistance,Traj_x,Traj_y,Traj_t,Traj_v,RefreshCounter);

% end function

== matlab function test_emplanner_cs/Audi_A8_Sedan_1/decision&planning module/EM Planner/calc path length and map between point and s ==
  data: trajectory_x input; path_s_end output; trajectory_y input; path_s output
function [path_s_end,path_s] = fcn(trajectory_x,trajectory_y)
% 该函数将计算以trajectory的s 与 x y 的对应关系，可以看作是trajectory index2s
n = length(trajectory_x);
path_s = zeros(n,1);
sum = 0;
for i = 2:length(trajectory_x)
    if isnan(trajectory_x(i))
        break;
    end
    sum = sum + sqrt((trajectory_x(i) - trajectory_x(i-1))^2 + (trajectory_y(i) - trajectory_y(i-1))^2);
    path_s(i) = sum;
end
% 计算出trajectory的长度
if i == n
    path_s_end = path_s(end);
else
    % 因为循环的退出条件为isnan(trajectory_x(i)) 所以 i 所对应的数为 nan 
    path_s_end = path_s(i - 1);
end

== matlab function test_emplanner_cs/Audi_A8_Sedan_1/decision&planning module/EM Planner/increase st point count ==
  data: s_init input; s output; s_dot_init input; s_dot2_init input; relative_time_init input; s_dot output; s_dot2 output; relative_time output
function [s,s_dot,s_dot2,relative_time] = fcn(s_init,s_dot_init,s_dot2_init,relative_time_init)
%该函数将增密s s_dot s_dot2
% 为什么需要增密，因为控制的执行频率是规划的10倍，轨迹点如果不够密，必然会导致规划效果不好
% 但是若在速度二次规划中点取的太多，会导致二次规划的矩阵规模太大计算太慢
% 所以方法是在二次规划中选取少量的点优化完毕后，在用此函数增密
T = relative_time_init(end);
n = 401;
dt = T/(n-1);
s = zeros(n,1);
s_dot = zeros(n,1);
s_dot2 = zeros(n,1);
relative_time = zeros(n,1);
for i = 1:n
    current_t = (i-1)*dt;
    for j = 1:length(relative_time_init)-1
        if relative_time_init(j) <= current_t && relative_time_init(j+1) > current_t
            break;
        end
    end
    x = current_t - relative_time_init(j);
    s(i) = s_init(j) + s_dot_init(j)*x + (1/3)*s_dot2_init(j)*x^2 + (1/6)*s_dot2_init(j+1)*x^2; 
    s_dot(i) = s_dot_init(j) + 0.5*s_dot2_init(j)*x + 0.5*s_dot2_init(j+1)*x;
    s_dot2(i) = s_dot2_init(j) + (s_dot2_init(j+1) - s_dot2_init(j))*x/(relative_time_init(j+1) - relative_time_init(j));
    relative_time(i) = current_t;
end

== matlab function test_emplanner_cs/Audi_A8_Sedan_1/decision&planning module/EM Planner/path and speed merge ==
  data: s input; trajectory_x output; s_dot input; s_dot2 input; relative_time input; current_time input; path_s input; trajectory_x_init input; trajectory_y_init input; trajectory_heading_init input; trajectory_kappa_init input; trajectory_y output; trajectory_heading output; trajectory_kappa output; trajectory_speed output; trajectory_accel output; trajectory_time output
function [trajectory_x,trajectory_y,trajectory_heading,trajectory_kappa,trajectory_speed,trajectory_accel,trajectory_time] = ...
    fcn(s,s_dot,s_dot2,relative_time,current_time,path_s,trajectory_x_init,trajectory_y_init,trajectory_heading_init,trajectory_kappa_init)
% 该函数将合并path和speed
% 由于path 是 60个点，speed 有 401个点，合并后，path和speed有401个点，因此需要做插值
n = 401;
trajectory_x = zeros(n,1);
trajectory_y = zeros(n,1);
trajectory_heading = zeros(n,1);
trajectory_kappa = zeros(n,1);
trajectory_speed = zeros(n,1);

trajectory_accel = zeros(n,1);
index = 1;
% 由于trajectory_x_init中不是所有的值都有效，(有nan) 所以要找到有效值的范围
while ~isnan(trajectory_x_init(index)) 
    index = index + 1;
end
index = index - 1;
trajectory_time = zeros(n,1);
for i = 1:n-1
    %interp1 线性插值
    % 若 x = [1,2] y = [3,4]
    %interp1(x,y,1.5) 会得到3.5
    %interp1 的缺点是 在端点或超过端点的，结果为nan
    % interp1(x,y,2) 不会等于4 而是会等于nan
    % interp1(x,y,6) 也会等于nan，所以在端点处要单独处理
    trajectory_x(i) = interp1(path_s(1:index),trajectory_x_init(1:index),s(i));
    trajectory_y(i) = interp1(path_s(1:index),trajectory_y_init(1:index),s(i));
    trajectory_heading(i) = interp1(path_s(1:index),trajectory_heading_init(1:index),s(i));
    trajectory_kappa(i) = interp1(path_s(1:index),trajectory_kappa_init(1:index),s(i));
    trajectory_time(i) = relative_time(i) + current_time;%速度规划会得到相对时间，转换成绝对时间
    trajectory_speed(i) = s_dot(i);
    trajectory_accel(i) = s_dot2(i);
end
% 端点单独处理
trajectory_x(end) = trajectory_x_init(end);
trajectory_y(end) = trajectory_y_init(end);
trajectory_heading(end) = trajectory_heading_init(end);
trajectory_kappa(end) = trajectory_kappa_init(end);
trajectory_time(end) = relative_time(end) + current_time;
trajectory_speed(end) = s_dot(end);
trajectory_accel(end) = s_dot2(end);

== matlab function test_emplanner_cs/Audi_A8_Sedan_1/decision&planning module/EM Planner/stitch trajectory ==
  data: trajectory_x input; trajectory_x_final output; trajectory_y input; trajectory_heading input; trajectory_kappa input; trajectory_speed input; trajectory_accel input; trajectory_time input; stitch_x input; stitch_y input; stitch_heading input; stitch_kappa input; stitch_speed input; stitch_accel input; stitch_time input; trajectory_y_final output; trajectory_heading_final output; trajectory_kappa_final output; trajectory_speed_final output; trajectory_accel_final output; trajectory_time_final output
function [trajectory_x_final,trajectory_y_final,trajectory_heading_final,trajectory_kappa_final,...
          trajectory_speed_final,trajectory_accel_final,trajectory_time_final] = fcn(trajectory_x,...
          trajectory_y,trajectory_heading,trajectory_kappa,trajectory_speed,trajectory_accel,trajectory_time,...
          stitch_x,stitch_y,stitch_heading,stitch_kappa,stitch_speed,stitch_accel,stitch_time)
% 轨迹拼接，把stitch trajectory 拼到规划完成的轨迹上
n = 401 + 20;
trajectory_x_final = zeros(n,1);
trajectory_y_final = zeros(n,1);
trajectory_heading_final = zeros(n,1);
trajectory_kappa_final = zeros(n,1);
trajectory_speed_final = zeros(n,1);
trajectory_accel_final = zeros(n,1);
trajectory_time_final = zeros(n,1);

trajectory_x_final = [stitch_x;trajectory_x];
trajectory_y_final = [stitch_y;trajectory_y];
trajectory_heading_final = [stitch_heading;trajectory_heading];
trajectory_kappa_final = [stitch_kappa;trajectory_kappa];
trajectory_speed_final = [stitch_speed;trajectory_speed];
trajectory_accel_final = [stitch_accel;trajectory_accel];
trajectory_time_final = [stitch_time;trajectory_time];

== matlab function test_emplanner_cs/Audi_A8_Sedan_1/decision&planning module/EM Planner/MATLAB Function1 ==
  data: qp_path_s input; qp_path_s_final output; qp_path_l input; qp_path_dl input; qp_path_ddl input; qp_path_l_final output; qp_path_dl_final output; qp_path_ddl_final output
function [qp_path_s_final,qp_path_l_final, qp_path_dl_final,qp_path_ddl_final] = fcn(qp_path_s,qp_path_l,qp_path_dl,qp_path_ddl)
% 该函数将增密qp_path
n_init = 20;
% 增密的点的个数
n = 501;
% 输出初始化
qp_path_s_final = zeros(n,1);
qp_path_l_final = zeros(n,1);
qp_path_dl_final = zeros(n,1);
qp_path_ddl_final = zeros(n,1);
ds = (qp_path_s(end) - qp_path_s(1))/(n-1);
index = 1;
for i = 1:n
    x = qp_path_s(1) + (i-1) * ds;
    qp_path_s_final(i) = x;
    while x >= qp_path_s(index)
        index = index + 1;
        if index == n_init
            break;
        end
    end
    % while 循环退出的条件是x<qp_path_s(index)，所以x对应的前一个s的编号是index-1 后一个编号是index
    pre = index - 1;
    cur = index;
    % 计算前一个点的l l' l'' ds 和后一个点的 l''
    delta_s = x - qp_path_s(pre);
    l_pre = qp_path_l(pre);
    dl_pre = qp_path_dl(pre);
    ddl_pre = qp_path_ddl(pre);
    ddl_cur = qp_path_ddl(cur);
    % 分段加加速度优化 
    qp_path_l_final(i) = l_pre + dl_pre * delta_s + (1/3)* ddl_pre * delta_s^2 + (1/6) * ddl_cur * delta_s^2;
    qp_path_dl_final(i) = dl_pre + 0.5 * ddl_pre * delta_s + 0.5 * ddl_cur * delta_s;
    qp_path_ddl_final(i) = ddl_pre + (ddl_cur - ddl_pre) * delta_s/(qp_path_s(cur) - qp_path_s(pre));
    %  因为此时x的后一个编号是index 必有x < qp_path_s(index),在下一个循环中x = x + ds 也未必大于
    %  qp_path_s(index)，这样就进入不了while循环，所以index 要回退一位
    index = index - 1;   
end

== matlab function test_emplanner_cs/Audi_A8_Sedan_1/control module/MATLAB Function ==
  data: trajectory_x input; xr output; trajectory_y input; trajectory_heading input; trajectory_kappa input; trajectory_speed input; trajectory_accel input; trajectory_time input; current_time input; yr output; thetar output; kappar output; vr output; ar output
function [xr,yr,thetar,kappar,vr,ar] = fcn(trajectory_x,trajectory_y,trajectory_heading,...
    trajectory_kappa,trajectory_speed,trajectory_accel,trajectory_time,current_time)
% 该函数根据规划的轨迹计算出期望跟踪的点
% 由于控制也是有延迟，所以控制发出的期望跟踪的点是current_time + 0.01;
control_time = current_time + 0.01;
% 规划发出的轨迹有一部分是拼接的，在刚启动的时候，stitch_time = -1,因此要先把它去掉
start_index = 1;
while (trajectory_time(start_index) == -1)
    start_index = start_index + 1;
end
% 使用interp1插值计算得到xr yr thetar,kappar,vr,ar
% 由于interp1在端点会得到nan，因此需要防一手
% 解释，为什么需要trajectory_time(start_index) ~= 0
% 因为在刚启动时规划先执行(100ms)，当规划完毕的时候控制已经执行了10次
% 那么在最开始的时候，规划还没给结果是控制已经执行了10次，在这10次中控制跟踪的轨迹是空轨迹
% simulink 空轨迹表示为 0，0，0，0，0，0......,这样trajectory_time
% 也全是0，trajectory_time不单调递增
% 而interp1(x,y,x0)要求x必须要单调递增，否则会报错，所以当规划首次运行时控制需要执行下面这个else分支的代码，否则会报错
if control_time > trajectory_time(start_index) && trajectory_time(start_index) ~= 0
    xr = interp1(trajectory_time(start_index:end),trajectory_x(start_index:end),control_time);
    yr = interp1(trajectory_time(start_index:end),trajectory_y(start_index:end),control_time);
    thetar = interp1(trajectory_time(start_index:end),trajectory_heading(start_index:end),control_time);
    kappar = interp1(trajectory_time(start_index:end),trajectory_kappa(start_index:end),control_time);
    vr = interp1(trajectory_time(start_index:end),trajectory_speed(start_index:end),control_time);
    ar = interp1(trajectory_time(start_index:end),trajectory_accel(start_index:end),control_time);
else
    xr = trajectory_x(start_index);
    yr = trajectory_y(start_index);
    thetar = trajectory_heading(start_index);
    kappar = trajectory_kappa(start_index);
    vr = trajectory_speed(start_index);
    ar = trajectory_accel(start_index);
end

== matlab function test_emplanner_cs/Audi_A8_Sedan_1/control module/control main/chassic steering system/MATLAB Function ==
  data: u input; right_steer output; la input; lb input
function right_steer = fcn(u,la,lb)
if abs(u)<1e-2
   right_steer = u;
else
   R =  (la+lb)/tan(u);
   right_steer = atan((la+lb)/(R+1.624/2));
end

== matlab function test_emplanner_cs/Audi_A8_Sedan_1/control module/control main/lateral control LQR/calc lqr K ==
  data: k1 input; k output; k2 input; k3 input; k4 input; vx input
function k  = fcn(k1,k2,k3,k4,vx)
    if abs(vx)<0.1
        k=[0,0,0,0];
    else
       
        k=[k1,k2,k3,k4];
    end
end

== matlab function test_emplanner_cs/Audi_A8_Sedan_1/control module/control main/lateral control LQR/err_kappa_calculate_module ==
  data: x input; y input; phi input; vx input; vy input; phi_dot input; xr input; yr input; thetar input; kappar input; err output; es output; s_dot output; phi output; projection_point_thetar output
function [err,es,s_dot,phi,projection_point_thetar] = fcn(x,y,phi,vx,vy,phi_dot,xr,yr,thetar,kappar)
    
    tor=[cos(thetar);sin(thetar)];
    nor=[-sin(thetar);cos(thetar)];
    d_err=[x-xr;y-yr];
    ed=nor'*d_err;
    es=tor'*d_err;
    %projection_point_thetar=thetar(dmin);%apollo
    projection_point_thetar=thetar+kappar*es;
    ed_dot=vy*cos(phi-projection_point_thetar)+vx*sin(phi-projection_point_thetar);
    %%%%%%%%%
    ephi=sin(phi-projection_point_thetar);
    %%%%%%%%%
    ss_dot=vx*cos(phi-projection_point_thetar)-vy*sin(phi-projection_point_thetar);
    s_dot=ss_dot/(1-kappar*ed);
    ephi_dot=phi_dot-kappar*s_dot;
    err=[ed;ed_dot;ephi;ephi_dot];
    
    
    
    
    
    
    
    
    
    
    
    


end

== matlab function test_emplanner_cs/Audi_A8_Sedan_1/control module/control main/lateral control LQR/feed_forword_control ==
  data: vx input; a input; forword_angle output; b input; m input; cf input; cr input; k input; kr input
function forword_angle = fcn(vx,a,b,m,cf,cr,k,kr)
    forword_angle=kr*(a+b-b*k(3)-(m*vx*vx/(a+b))*((b/cf)+(a/cr)*k(3)-(a/cr)));
end

== matlab function test_emplanner_cs/Audi_A8_Sedan_1/decision&planning module/EM Planner/generate convex space ==
  data: dp_path_s input; l_min output; dp_path_l input; static_obs_s_set input; static_obs_l_set input; static_obs_length input; static_obs_width input; l_max output
function [l_min,l_max] = fcn(dp_path_s,dp_path_l,static_obs_s_set,static_obs_l_set,static_obs_length,static_obs_width)
%该函数将输出每个离散的dp_path_s的点的s所对应的l边界l_min,l_max
%输入为： 动态规划的曲线dp_path_s dp_path_l
          %障碍物中心点的坐标static_obs_s_set,static_obs_l_set
          %障碍物的长宽static_obs_length,static_obs_width
%输出为：l_min,l_max的上下界
%一般真实障碍物投影到frenet坐标后，长宽会变得扭曲，近似用直角坐标的代替
%所以em planner 不能处理参考线曲率过大的场景（r>200）
%大曲率的避障，参考线模块，障碍物模块，速度规划模块要做特殊处理
%输出初始化，如果无障碍l的边界默认为+_6
l_min=ones(60,1)*-6;
l_max=ones(60,1)*6;
%对每个障碍物做遍历
for i=1:length(static_obs_s_set)
    if isnan(static_obs_s_set(i))
        break;
    end
    %计算障碍物头部和尾部s
    obs_s_min=static_obs_s_set(i)-static_obs_length/2;
    obs_s_max=static_obs_s_set(i)+static_obs_length/2;
    %找到obs_s_min,obs_s_max在dp_path_s中的位置
    start_index=FindNearIndex(dp_path_s,obs_s_min);
    end_index=FindNearIndex(dp_path_s,obs_s_max);
    %判断dp_path_l在障碍物的上面还是下面，path在obs上面即决策为向左绕，否则为向右绕
    centre_index=FindNearIndex(dp_path_s,static_obs_s_set(i));
    if start_index==1&&end_index==1
        %障碍物已经在host后面
        continue;
    end
    path_l=dp_path_l(centre_index);
    if path_l>static_obs_l_set(i)
        %意味着决策为向左绕过障碍物
        for j=start_index:end_index
            %l_min(j)为所有决策为向左绕过障碍物的l边界的最大值
            l_min(j)=max(l_min(j),static_obs_l_set(i)+static_obs_width/2);
        end
    else
    %意味着决策为向右绕过障碍物
        for j=start_index:end_index
            %l_max(j)为所有决策为向右绕过障碍物的l边界的最小值
            l_max(j)=min(l_max(j),static_obs_l_set(i)-static_obs_width/2);
        end
    end
end

function y=FindNearIndex(dp_path_s,obs_s)
%该函数将找到dp_path_s上的所有点中，与obs_s最近的点，并返回该点在dp_path_s的编号
%dp_path_s上的点是动态规划的结果，必然大于0，小于60
%obs_s是障碍物在整个referenceline上投影所得的坐标，所以obs_s有可能小于0，也有可能大于59
if dp_path_s(1)>=obs_s
    %障碍物在车的后面
    y=1;
    return;
elseif dp_path_s(end)<obs_s
    %障碍物在车的前面过远
    y=60;
    return;
else
    index=1;
    while dp_path_s(index)<obs_s
        index=index+1;
    end
    if dp_path_s(index)-obs_s>obs_s-dp_path_s(index-1)
        y=index-1;
    else
        y=index;
    end
end

== matlab function test_emplanner_cs/Audi_A8_Sedan_1/control module/control main/lateral control LQR/feedback_control+feedforword_control ==
  data: k input; angle output; err input; forword_angle input
function angle = fcn(k,err,forword_angle)

    angle=-k*err+forword_angle;
end

== matlab function test_emplanner_cs/Audi_A8_Sedan_1/control module/control main/lateral control LQR/predict_module ==
  data: x input; pred_x_ctrl output; y input; phi input; vx input; vy input; phi_dot input; ts input; pred_y_ctrl output; pred_yaw_ctrl output; pred_vx_ctrl output; pred_vy_ctrl output; pred_yaw_dot_ctrl output
function [pred_x_ctrl,pred_y_ctrl,pred_yaw_ctrl,pred_vx_ctrl,pred_vy_ctrl,pred_yaw_dot_ctrl] = fcn(x,y,phi,vx,vy,phi_dot,ts)
    pred_x_ctrl=x+vx*ts*cos(phi)-vy*ts*sin(phi);
    pred_y_ctrl=y+vy*ts*cos(phi)+vx*ts*sin(phi);
    pred_yaw_ctrl=phi;
    pred_vx_ctrl=vx;
    pred_vy_ctrl=vy;
    pred_yaw_dot_ctrl=phi_dot;
end

== matlab function test_emplanner_cs/Audi_A8_Sedan_1/decision&planning module/EM Planner/calc speed planning start condition ==
  data: plan_start_vx input; plan_start_s_dot output; plan_start_vy input; plan_start_ax input; plan_start_ay input; plan_start_heading input; plan_start_s_dot2 output
function [plan_start_s_dot,plan_start_s_dot2] = fcn(plan_start_vx,plan_start_vy,plan_start_ax,plan_start_ay,plan_start_heading)
% 该函数计算速度规划的初始条件
tor = [cos(plan_start_heading);sin(plan_start_heading)];
v_t = tor'*[plan_start_vx;plan_start_vy];
a_t = tor'*[plan_start_ax;plan_start_ay];
plan_start_s_dot = v_t;
plan_start_s_dot2 = a_t;

== matlab function test_emplanner_cs/Audi_A8_Sedan_1/decision&planning module/EM Planner/simple speed qp planning ==
  data: plan_start_s_dot input; s_init output; plan_start_s_dot2 input; s_end input; recommend_T input; s_dot_init output; s_dot2_init output; relative_time_init output
function [s_init,s_dot_init,s_dot2_init,relative_time_init] = fcn(plan_start_s_dot,plan_start_s_dot2,s_end,recommend_T)
%简单速度二次规划
coder.extrinsic("quadprog")
n = 51;
s_init = zeros(n,1);
s_dot_init = zeros(n,1);
s_dot2_init = zeros(n,1);
relative_time_init = zeros(n,1);

Aeq = zeros(3*n,2*n - 2);
beq = zeros(2*n - 2,1);
lb = ones(3*n,1);
ub = lb;
dt = recommend_T/(n-1);
A_sub =[1,0;
        dt,1;
        (1/3)*dt^2,(1/2)*dt;
        -1,0;
        0,-1;
        (1/6)*dt^2,dt/2];
for i = 1:n - 1
    Aeq(3*i-2:3*i+3,2*i-1:2*i) = A_sub;
end

for i = 1:n
   lb(3*i - 2) = -inf;
   lb(3*i - 1) = 0;
   lb(3*i) = -8;
   ub(3*i - 2) = inf;
   ub(3*i - 1) = 50;
   ub(3*i) = 2;
end
lb(1) = 0;
lb(2) = plan_start_s_dot;
lb(3) = plan_start_s_dot2;
ub(1) = lb(1);
ub(2) = lb(2);
ub(3) = lb(3);
lb(3*n - 2) = s_end;
ub(3*n - 2) = s_end;
A3 = zeros(3*n,3*n);
A4 = zeros(3*n,n - 1);
A4_sub =[0;0;1;0;0;-1];
for i = 1:n - 1
   A3(3*i,3*i) = 1;
   A4(3*i-2:3*i+3,i:i) = A4_sub;
end
A3(3*n,3*n) = 1;
H = A3 + 100*(A4*A4');
H = 2*H;
f = zeros(3*n,1);
X = quadprog(H,f,[],[],Aeq',beq,lb,ub);
for i = 1:n
   s_init(i) = X(3*i - 2);
   s_dot_init(i) = X(3*i - 1);
   s_dot2_init(i) = X(3*i);
   relative_time_init(i) = (i - 1)*dt;
end

== matlab function test_emplanner_cs/Audi_A8_Sedan_1/control module/control main/longitudinal control double PID/MATLAB Function1 ==
  data: u input; throttle output; brake output
function [throttle,brake] = fcn(u)
    if u>=0
        throttle=u;
        brake=0;
    else
        throttle=0;
        brake=-u;
    end

== matlab function test_emplanner_cs/Audi_A8_Sedan_2/PathFollower_Preview_1/LateralController/CTRL REFERENCES/Find Reference Point (pref0) on Trajectory closest to P0 Point (p0)/eml_find_closest_trajectory_points0 ==
  data: pvp input size=2; Actor_traj_distance output; TrajOffset_x_y_Y input size=3; ActorOffset_Left_Right input; p0 input size=3; Traj_x parameter; Traj_y parameter; Actor_traj_angle output; RefreshCounter parameter
function [Actor_traj_distance,Actor_traj_angle]  = eml_find_closest_trajectory_points0(pvp,TrajOffset_x_y_Y,ActorOffset_Left_Right,p0,Traj_x,Traj_y,RefreshCounter)

[Actor_traj_distance,Actor_traj_angle]  = emlfcn_find_closest_trajectory_points0(pvp,TrajOffset_x_y_Y,ActorOffset_Left_Right,p0,Traj_x,Traj_y,RefreshCounter);

% end function
